simulink model "Thermoelectric_cooling"  (R2019a)
settings: Solver=VariableStepAuto  StartTime=0.0  StopTime=10.0  RelTol=1e-3
settings Model: Creator=student  LastModifiedBy=student

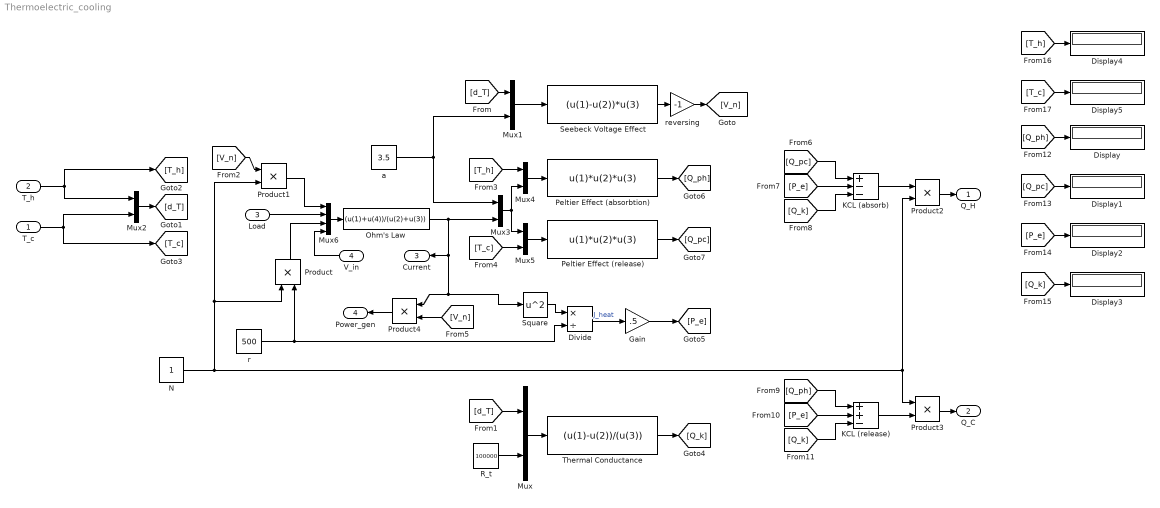
== system Thermoelectric_cooling ==
  T_c : Inport
  "T_h " : Inport  Port=2
  Load : Inport  Port=3
  "V_in " : Inport  Port=4
  Display{,1..5} (6 alike) : Display
  Divide : Product  Inputs=*/
  Gain : Gain  Gain=.5
  KCL (absorb) : Sum  Inputs=+--
  KCL (release) : Sum  Inputs=++-
  Mux{,1..5} (6 alike) : Mux  Inputs=2
  Mux6 : Mux
  N : Constant
  Ohm's Law : Fcn  Expr=(u(1)+u(4))/(u(2)+u(3))
  Peltier Effect (absorbtion) : Fcn  Expr=u(1)*u(2)*u(3)
  Peltier Effect (release) : Fcn  Expr=u(1)*u(2)*u(3)
  Product{,1..4} (5 alike) : Product
  "R_t " : Constant  Value=100000
  Seebeck Voltage Effect : Fcn  Expr=(u(1)-u(2))*u(3)
  Square : Math  Operator=square  SaturateOnIntegerOverflow=on
  Thermal Conductance : Fcn  Expr=(u(1)-u(2))/(u(3))
  a : Constant  Value=3.5
  r : Constant  Value=500
  "reversing " : Gain  Gain=-1
  Q_H : Outport
  Q_C : Outport  Port=2
  Current : Outport  Port=3
  Power_gen : Outport  Port=4
  wires:
  [Q_ph] -> KCL (release)/1
  Mux6/1 -> Ohm's Law/1
  Mux5/1 -> Peltier Effect (release)/1
  KCL (release)/1 -> Product3/2
  [Q_k] -> KCL (absorb)/3
  [Q_k] -> KCL (release)/3
  [V_n] -> Product1/1
  Product/1 -> Mux6/3
  [P_e] -> KCL (absorb)/2
  Mux3/1 -> Mux5/1, Mux4/2
  Mux1/1 -> Seebeck Voltage Effect/1
  N/1 -> Product2/2, Product3/1, Product1/2, Product/1
  "V_in "/1 -> Mux6/4
  r/1 -> Product/2, Divide/2
  Peltier Effect (release)/1 -> [Q_pc]
  Square/1 -> Divide/1
  Gain/1 -> [P_e]
  Product3/1 -> Q_C/1
  Load/1 -> Mux6/2
  Mux/1 -> Thermal Conductance/1
  [d_T] -> Mux1/1
  [P_e] -> KCL (release)/2
  Mux2/1 -> [d_T]
  a/1 -> Mux1/2, Mux3/1
  Thermal Conductance/1 -> [Q_k]
  KCL (absorb)/1 -> Product2/1
  Product2/1 -> Q_H/1
  Mux4/1 -> Peltier Effect (absorbtion)/1
  [d_T] -> Mux/1
  "R_t "/1 -> Mux/2
  [Q_pc] -> KCL (absorb)/1
  [T_h] -> Mux4/1
  Peltier Effect (absorbtion)/1 -> [Q_ph]
  [T_c] -> Mux5/2
  Product1/1 -> Mux6/1
  Divide/1 -> Gain/1  "J_heat"
  T_c/1 -> Mux2/2, [T_c]
  "T_h "/1 -> Mux2/1, [T_h]
  Product4/1 -> Power_gen/1
  Ohm's Law/1 -> Mux3/2, Square/1, Product4/1, Current/1
  [Q_ph] -> Display/1
  [P_e] -> Display2/1
  [Q_k] -> Display3/1
  [Q_pc] -> Display1/1
  [T_c] -> Display5/1
  [T_h] -> Display4/1
  Seebeck Voltage Effect/1 -> "reversing "/1
  "reversing "/1 -> [V_n]
  [V_n] -> Product4/2
